simulink model "s_c856m4k"  (R2016b)
settings: Solver=VariableStepAuto  StartTime=0.0  StopTime=10  RelTol=1e-3  EnableMultiTasking=on
undefined symbols (not defined in the file): fft_stages
libraries: xbsIndex_r4 x11811, casper_library_misc x54, casper_library_scopes x5, xps_library x2
(part 10 of 92)

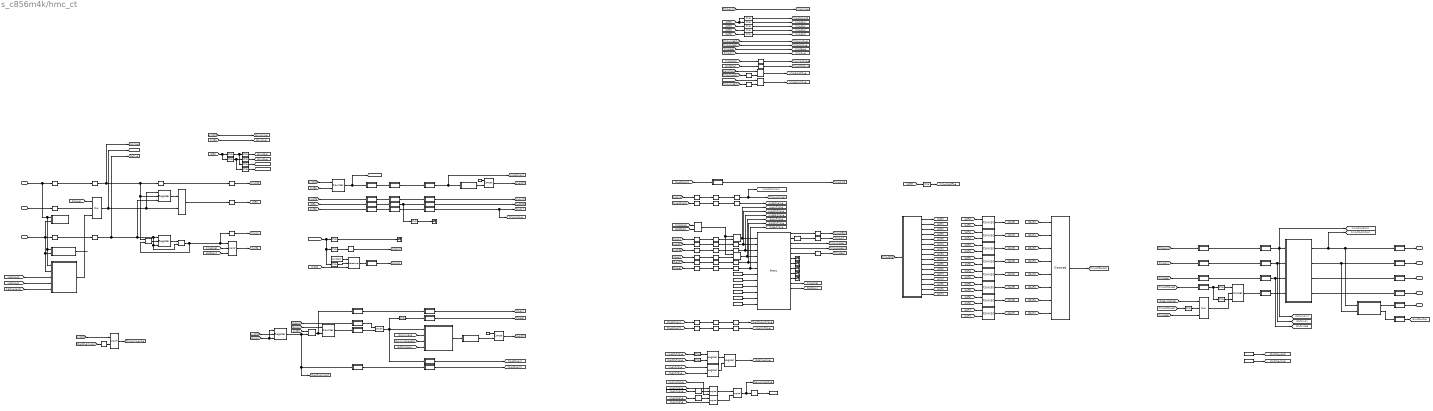
== system s_c856m4k/hmc_ct ==
  note: Sync debugging
  note: Map writes across HMC
      | for performance.
  note: Write two successive words together.
  note: Write is linear.
  note: Read when write switches banks.
  note: Map the output read to collect like channels.
  note: Map writes across HMC
      | for performance.
  note: TVG
  note: Eight parallel channels.
  note: Double buffer the data to form output packets
  note: HMC
  note: Check for _en sync and bank errors
  in_sync : Inport
  in_dv : Inport  Port=2
  in_d128 : Inport  Port=3
  Assertion : Assertion
  Concat{,1..10,12} (12 alike) : xbsIndex_r4/Concat  num_inputs=2  dbl_ovrd=off  block_type=concat
  Concat11 : xbsIndex_r4/Concat  num_inputs=8  dbl_ovrd=off  block_type=concat
  Concat13 : xbsIndex_r4/Concat  num_inputs=3  dbl_ovrd=off  block_type=concat
  Constant : xbsIndex_r4/Constant  const=2^((input_len_bits - 1) + output_len_bits + 1) - 1  gui_display_data_type=Fixed-point  arith_type=Unsigned  n_bits=(input_len_bits - 1) + output_len_bits  bin_pt=0  preci_type=Single  exp_width=8  frac_width=24  explicit_period=on  period=1  equ=P=C  opselect=C  inp2=PCIN>>17  opr=+  inp1=P  carry=CIN  dbl_ovrd=off  block_type=constant
  Constant1 : xbsIndex_r4/Constant  const=0  gui_display_data_type=Boolean  arith_type=Boolean  n_bits=1  bin_pt=0  preci_type=Single  exp_width=8  frac_width=24  explicit_period=on  period=1  equ=P=C  opselect=C  inp2=PCIN>>17  opr=+  inp1=P  carry=CIN  dbl_ovrd=off  block_type=constant
  Constant16 : xbsIndex_r4/Constant  const=384  gui_display_data_type=Fixed-point  arith_type=Unsigned  n_bits=9  bin_pt=0  preci_type=Single  exp_width=8  frac_width=24  explicit_period=on  period=1  equ=P=C  opselect=C  inp2=PCIN>>17  opr=+  inp1=P  carry=CIN  dbl_ovrd=off  block_type=constant
  Constant17 : xbsIndex_r4/Constant  const=128  gui_display_data_type=Fixed-point  arith_type=Unsigned  n_bits=9  bin_pt=0  preci_type=Single  exp_width=8  frac_width=24  explicit_period=on  period=1  equ=P=C  opselect=C  inp2=PCIN>>17  opr=+  inp1=P  carry=CIN  dbl_ovrd=off  block_type=constant
  Constant2 : xbsIndex_r4/Constant  const=0  gui_display_data_type=Fixed-point  arith_type=Unsigned  n_bits=27  bin_pt=0  preci_type=Single  exp_width=8  frac_width=24  explicit_period=on  period=1  equ=P=C  opselect=C  inp2=PCIN>>17  opr=+  inp1=P  carry=CIN  dbl_ovrd=off  block_type=constant
  Constant3 : xbsIndex_r4/Constant  const=0  gui_display_data_type=Fixed-point  arith_type=Unsigned  n_bits=256  bin_pt=0  preci_type=Single  exp_width=8  frac_width=24  explicit_period=on  period=1  equ=P=C  opselect=C  inp2=PCIN>>17  opr=+  inp1=P  carry=CIN  dbl_ovrd=off  block_type=constant
  Constant4 : xbsIndex_r4/Constant  const=0  gui_display_data_type=Fixed-point  arith_type=Unsigned  n_bits=9  bin_pt=0  preci_type=Single  exp_width=8  frac_width=24  explicit_period=on  period=1  equ=P=C  opselect=C  inp2=PCIN>>17  opr=+  inp1=P  carry=CIN  dbl_ovrd=off  block_type=constant
  Constant5 : xbsIndex_r4/Constant  const=0  gui_display_data_type=Boolean  arith_type=Boolean  n_bits=1  bin_pt=0  preci_type=Single  exp_width=8  frac_width=24  explicit_period=on  period=1  equ=P=C  opselect=C  inp2=PCIN>>17  opr=+  inp1=P  carry=CIN  dbl_ovrd=off  block_type=constant
  Constant6 : xbsIndex_r4/Constant  const=0  gui_display_data_type=Fixed-point  arith_type=Unsigned  n_bits=27 - (input_len_bits + output_len_bits)  bin_pt=0  preci_type=Single  exp_width=8  frac_width=24  explicit_period=on  period=1  equ=P=C  opselect=C  inp2=PCIN>>17  opr=+  inp1=P  carry=CIN  dbl_ovrd=off  block_type=constant
  Constant7 : xbsIndex_r4/Constant  const=0  gui_display_data_type=Fixed-point  arith_type=Unsigned  n_bits=27  bin_pt=0  preci_type=Single  exp_width=8  frac_width=24  explicit_period=on  period=1  equ=P=C  opselect=C  inp2=PCIN>>17  opr=+  inp1=P  carry=CIN  dbl_ovrd=off  block_type=constant
  Constant8 : xbsIndex_r4/Constant  const=0  gui_display_data_type=Fixed-point  arith_type=Unsigned  n_bits=27 - (input_len_bits + output_len_bits)  bin_pt=0  preci_type=Single  exp_width=8  frac_width=24  explicit_period=on  period=1  equ=P=C  opselect=C  inp2=PCIN>>17  opr=+  inp1=P  carry=CIN  dbl_ovrd=off  block_type=constant
  Delay{1..2,4..13,16..19,21..23,25..27,30..32,41} (26 alike) : xbsIndex_r4/Delay  rst=off  infoeditControl=Selection of Reset will increase slice count due to use of real FFs and instead of SRLs  en=off  latency=1  reg_retiming=off  dbl_ovrd=off  block_type=delay
      settings: infoedit=Hardware notes: A delay line is a chain, each link of which is an SRL16 or SRL32 followed by a flip-flop.
  Delay{14..15,35,39,42} (5 alike) : xbsIndex_r4/Delay  rst=off  infoeditControl=Selection of Reset will increase slice count due to use of real FFs and instead of SRLs  en=off  latency=2  reg_retiming=off  dbl_ovrd=off  block_type=delay
      settings: infoedit=Hardware notes: A delay line is a chain, each link of which is an SRL16 or SRL32 followed by a flip-flop.
  Delay{3,20,24,28..29,37..38,40} (8 alike) : xbsIndex_r4/Delay  rst=off  infoeditControl=Selection of Reset will increase slice count due to use of real FFs and instead of SRLs  en=off  latency=5  reg_retiming=off  dbl_ovrd=off  block_type=delay
      settings: infoedit=Hardware notes: A delay line is a chain, each link of which is an SRL16 or SRL32 followed by a flip-flop.
  Delay33 : xbsIndex_r4/Delay  rst=off  infoeditControl=Selection of Reset will increase slice count due to use of real FFs and instead of SRLs  en=off  latency=4  reg_retiming=off  dbl_ovrd=off  block_type=delay
      settings: infoedit=Hardware notes: A delay line is a chain, each link of which is an SRL16 or SRL32 followed by a flip-flop.
  Delay34 : xbsIndex_r4/Delay  rst=off  infoeditControl=Selection of Reset will increase slice count due to use of real FFs and instead of SRLs  en=off  latency=4  reg_retiming=off  dbl_ovrd=off  block_type=delay
      settings: infoedit=Hardware notes: A delay line is a chain, each link of which is an SRL16 or SRL32 followed by a flip-flop.
  Delay36 : xbsIndex_r4/Delay  rst=off  infoeditControl=Selection of Reset will increase slice count due to use of real FFs and instead of SRLs  en=off  latency=4  reg_retiming=off  dbl_ovrd=off  block_type=delay
      settings: infoedit=Hardware notes: A delay line is a chain, each link of which is an SRL16 or SRL32 followed by a flip-flop.
  Inverter{,1..2,4..6} (6 alike) : xbsIndex_r4/Inverter  en=off  latency=0  dbl_ovrd=off  block_type=inv
  Inverter3 : xbsIndex_r4/Inverter  en=off  latency=1  dbl_ovrd=off  block_type=inv
  Logical : xbsIndex_r4/Logical  logical_function=AND  inputs=2  en=off  latency=0  precision=Full  arith_type=Unsigned  n_bits=16  bin_pt=0  align_bp=on  dbl_ovrd=off  block_type=logical
  Logical1 : xbsIndex_r4/Logical  logical_function=AND  inputs=2  en=off  latency=1  precision=User Defined  arith_type=Boolean  n_bits=1  bin_pt=0  align_bp=on  dbl_ovrd=off  block_type=logical
  Logical10 : xbsIndex_r4/Logical  logical_function=OR  inputs=2  en=off  latency=0  precision=Full  arith_type=Unsigned  n_bits=16  bin_pt=0  align_bp=on  dbl_ovrd=off  block_type=logical
  Logical{5,7,11,13} (4 alike) : xbsIndex_r4/Logical  logical_function=AND  inputs=2  en=off  latency=5  precision=Full  arith_type=Unsigned  n_bits=16  bin_pt=0  align_bp=on  dbl_ovrd=off  block_type=logical
  Logical12 : xbsIndex_r4/Logical  logical_function=AND  inputs=2  en=off  latency=1  precision=User Defined  arith_type=Boolean  n_bits=1  bin_pt=0  align_bp=on  dbl_ovrd=off  block_type=logical
  Logical14 : xbsIndex_r4/Logical  logical_function=OR  inputs=2  en=off  latency=5  precision=Full  arith_type=Unsigned  n_bits=16  bin_pt=0  align_bp=on  dbl_ovrd=off  block_type=logical
  Logical15 : xbsIndex_r4/Logical  logical_function=AND  inputs=2  en=off  latency=2  precision=Full  arith_type=Unsigned  n_bits=16  bin_pt=0  align_bp=on  dbl_ovrd=off  block_type=logical
  Logical2 : xbsIndex_r4/Logical  logical_function=OR  inputs=2  en=off  latency=0  precision=Full  arith_type=Unsigned  n_bits=16  bin_pt=0  align_bp=on  dbl_ovrd=off  block_type=logical
  Logical3 : xbsIndex_r4/Logical  logical_function=AND  inputs=2  en=off  latency=0  precision=Full  arith_type=Unsigned  n_bits=16  bin_pt=0  align_bp=on  dbl_ovrd=off  block_type=logical
  Logical4 : xbsIndex_r4/Logical  logical_function=AND  inputs=2  en=off  latency=1  precision=Full  arith_type=Unsigned  n_bits=16  bin_pt=0  align_bp=on  dbl_ovrd=off  block_type=logical
  Logical6 : xbsIndex_r4/Logical  logical_function=AND  inputs=2  en=on  latency=5  precision=Full  arith_type=Unsigned  n_bits=16  bin_pt=0  align_bp=on  dbl_ovrd=off  block_type=logical
  Logical8 : xbsIndex_r4/Logical  logical_function=AND  inputs=2  en=off  latency=0  precision=Full  arith_type=Unsigned  n_bits=16  bin_pt=0  align_bp=on  dbl_ovrd=off  block_type=logical
  Logical9 : xbsIndex_r4/Logical  logical_function=AND  inputs=3  en=off  latency=2  precision=Full  arith_type=Unsigned  n_bits=16  bin_pt=0  align_bp=on  dbl_ovrd=off  block_type=logical
  Mux : xbsIndex_r4/Mux  inputs=2  en=off  latency=2  precision=Full  arith_type=Unsigned  n_bits=16  bin_pt=14  quantization=Truncate  overflow=Wrap  dbl_ovrd=off  block_type=mux
  Mux3 : xbsIndex_r4/Mux  inputs=2  en=off  latency=2  precision=Full  arith_type=Unsigned  n_bits=16  bin_pt=14  quantization=Truncate  overflow=Wrap  dbl_ovrd=off  block_type=mux
  Register : xbsIndex_r4/Register  init=0  rst=on  en=on  dbl_ovrd=off  block_type=register
  Relational1 : xbsIndex_r4/Relational  mode=a=b  op_type=Bool  en=on  latency=1  dbl_ovrd=off  block_type=relational
  Slice : xbsIndex_r4/Slice  nbits=12  boolean_output=off  mode=Lower Bit Location + Width  bit1=0  base1=MSB of Input  bit0=0  base0=LSB of Input  dbl_ovrd=off  block_type=slice
  Slice1 : xbsIndex_r4/Slice  nbits=9  boolean_output=off  mode=Lower Bit Location + Width  bit1=0  base1=MSB of Input  bit0=0  base0=LSB of Input  dbl_ovrd=off  block_type=slice
  Slice12 : xbsIndex_r4/Slice  nbits=1  boolean_output=on  mode=Lower Bit Location + Width  bit1=0  base1=MSB of Input  bit0=input_len_bits - 1 + output_len_bits  base0=LSB of Input  dbl_ovrd=off  block_type=slice
  Slice13 : xbsIndex_r4/Slice  nbits=1  boolean_output=on  mode=Lower Bit Location + Width  bit1=0  base1=MSB of Input  bit0=input_len_bits - 1 + output_len_bits  base0=LSB of Input  dbl_ovrd=off  block_type=slice
  Slice{2..5} (4 alike) : xbsIndex_r4/Slice  nbits=input_len_bits + 2  boolean_output=off  mode=Lower Bit Location + Width  bit1=0  base1=MSB of Input  bit0=0  base0=LSB of Input  dbl_ovrd=off  block_type=slice
  Slice6 : xbsIndex_r4/Slice  nbits=input_len_bits + 2  boolean_output=on  mode=Upper Bit Location + Width  bit1=0  base1=MSB of Input  bit0=0  base0=LSB of Input  dbl_ovrd=off  block_type=slice
  Terminator{1,16,20..24} (7 alike) : Terminator
  bank : xbsIndex_r4/Slice  nbits=1  boolean_output=on  mode=Upper Bit Location + Width  bit1=0  base1=MSB of Input  bit0=0  base0=LSB of Input  dbl_ovrd=off  block_type=slice
  bank1 : xbsIndex_r4/Slice  nbits=12  boolean_output=off  mode=Upper Bit Location + Width  bit1=-4  base1=MSB of Input  bit0=0  base0=LSB of Input  dbl_ovrd=off  block_type=slice
  bank2 : xbsIndex_r4/Slice  nbits=12  boolean_output=off  mode=Upper Bit Location + Width  bit1=-4  base1=MSB of Input  bit0=128  base0=LSB of Input  dbl_ovrd=off  block_type=slice
  bank3 : xbsIndex_r4/Slice  nbits=12  boolean_output=off  mode=Upper Bit Location + Width  bit1=-4  base1=MSB of Input  bit0=128  base0=LSB of Input  dbl_ovrd=off  block_type=slice
  bank4 : xbsIndex_r4/Slice  nbits=128  boolean_output=off  mode=Lower Bit Location + Width  bit1=0  base1=MSB of Input  bit0=128  base0=LSB of Input  dbl_ovrd=off  block_type=slice
  bank5 : xbsIndex_r4/Slice  nbits=128  boolean_output=off  mode=Lower Bit Location + Width  bit1=0  base1=MSB of Input  bit0=0  base0=LSB of Input  dbl_ovrd=off  block_type=slice
  bank6 : xbsIndex_r4/Slice  nbits=12  boolean_output=on  mode=Upper Bit Location + Width  bit1=0  base1=MSB of Input  bit0=128  base0=LSB of Input  dbl_ovrd=off  block_type=slice
  bank7 : xbsIndex_r4/Slice  nbits=12  boolean_output=on  mode=Upper Bit Location + Width  bit1=0  base1=MSB of Input  bit0=128  base0=LSB of Input  dbl_ovrd=off  block_type=slice
  bus_expand1 : Subsystem  AncestorBlock=casper_library_flow_control/bus_expand  mask(bus_expand){mode=divisions of equal size, outputNum=16, outputWidth=16, outputBinaryPt=0, outputArithmeticType=0, show_format=off, outputToWorkspace=off, variablePrefix=out, outputToModelAsWell=on}
      mask prompts: outputNum "Number of outputs:"; outputWidth "Output width:"; outputBinaryPt "Output binary point position:"; outputArithmeticType "Output arithmetic type (ufix=0, fix=1, bool=2):"; show_format "Print format string?"; outputToWorkspace "Output to workspace?"; variablePrefix "Variable name prefix:"; outputToModelAsWell "Output to model as well?"
      mask help:
      | Expands a 'bus' made using a bus_create or Xilinx
      | concat block.
      | The input will be divided into the specified number
      | of outputs with the specified arithmetic types.
      | Divisions are made from most significant bit.
      mask init: same as s_c856m4k/bus_expand
      settings: AttributesFormatString=16 outputs
      mask TypeOptions mode: divisions of equal size | divisions of arbitrary size
      mask Callback mode: bus_expand_callback();
      mask Callback outputWidth: bus_expand_callback();
      mask Callback outputToWorkspace: bus_expand_callback();
  convert_rd_en4 : xbsIndex_r4/Convert  gui_display_data_type=Boolean  arith_type=Boolean  n_bits=128  bin_pt=0  float_type=Single  exp_bits=8  fraction_bits=24  quantization=Truncate  overflow=Wrap  en=off  latency=0  pipeline=off  dbl_ovrd=off  block_type=convert
      settings: xl_area=[0, 0, 0, 0, 0, 0, 0]
  edge_detect1 : Subsystem  AncestorBlock=casper_library_misc/edge_detect  mask(edge_detect){edge=Rising, polarity=Active High, x_in=[0 0.08 0.08 0.16 0.16 0.24 0.24 0.32 0.32 0.4], y_in=[-1 -1  1  1  1  1  1  1  1  1], x_out=[0.6 0.68 0.68 0.76 0.76 0.84 0.84 0.92 0.92 1], y_out=[-1 -1  1  1 -1 -1 -1 -1 -1 -1]}
      mask prompts: edge "Edge Type"; polarity "Output Polarity"; x_in "Input X Positions"; y_in "Input Y Positions"; x_out "Output X Positions"; y_out "Output Y Positions"
      mask help: Output is active for one-cycle after each edge of the specified type (i.e. rising, falling or both).
      mask init: same as s_c856m4k/edge_detect1
      settings: AttributesFormatString=|
      | rising edges
      | active high
      mask Help: Output is active for one-cycle after each edge of the specified type (i.e. rising, falling, or both).  Latency is zero.
      mask TypeOptions edge: Rising | Falling | Both
      mask TypeOptions polarity: Active High | Active Low
      mask Display:
      | plot(x_in_num,0.5+y_in_num*0.2);
      | plot(x_out_num,0.5+y_out_num*0.2);
  edge_detect2 : Subsystem  AncestorBlock=casper_library_misc/edge_detect  mask(edge_detect){edge=Rising, polarity=Active High, x_in=[0 0.08 0.08 0.16 0.16 0.24 0.24 0.32 0.32 0.4], y_in=[-1 -1  1  1  1  1  1  1  1  1], x_out=[0.6 0.68 0.68 0.76 0.76 0.84 0.84 0.92 0.92 1], y_out=[-1 -1  1  1 -1 -1 -1 -1 -1 -1]}
      mask prompts: edge "Edge Type"; polarity "Output Polarity"; x_in "Input X Positions"; y_in "Input Y Positions"; x_out "Output X Positions"; y_out "Output Y Positions"
      mask help: Output is active for one-cycle after each edge of the specified type (i.e. rising, falling or both).
      mask init: same as s_c856m4k/edge_detect1
      settings: AttributesFormatString=|
      | rising edges
      | active high
      mask Help: Output is active for one-cycle after each edge of the specified type (i.e. rising, falling, or both).  Latency is zero.
      mask TypeOptions edge: Rising | Falling | Both
      mask TypeOptions polarity: Active High | Active Low
      mask Display:
      | plot(x_in_num,0.5+y_in_num*0.2);
      | plot(x_out_num,0.5+y_out_num*0.2);
  hmc : xps_library/hmc  Tag=xps:hmc  mez=0  sim_depth=(input_len_bits-1) + output_len_bits + 1  sim_latency=5  sim_rand=on
  hmc_addr_opt : Subsystem
  hmc_addr_opt1 : Subsystem
  last_tag2 : xbsIndex_r4/Register  init=0  rst=on  en=on  dbl_ovrd=off  block_type=register
  make_interleaved_freqs : Subsystem  mask{chan_bits=12, xeng_bits=4}
      mask prompts: chan_bits "Number of channels (2^?)"; xeng_bits "Number of x-engines (2^?)"
  obuf : Subsystem  mask{output_vec_bits=output_len_bits, pkt_buffer_latency=10, omux_latency=15}
      mask prompts: output_vec_bits "CT output vector bits"; pkt_buffer_latency "Output buffer latency"; omux_latency "Output mux latency"
  prev_word : xbsIndex_r4/Register  init=0  rst=on  en=on  dbl_ovrd=off  block_type=register
  rd_addr_ctr : xbsIndex_r4/Counter  cnt_type=Free Running  cnt_to=Inf  operation=Up  start_count=0  cnt_by_val=1  arith_type=Unsigned  n_bits=input_len_bits - 1 + output_len_bits  bin_pt=0  load_pin=off  rst=on  en=on  explicit_period=on  period=1  use_behavioral_HDL=off  implementation=Fabric  dbl_ovrd=off  block_type=counter
  read_map_gen_interleave : Subsystem  mask{in_vec_bits=input_len_bits - 1, out_vec_bits=output_len_bits}
      mask prompts: in_vec_bits "Input vector bits"; out_vec_bits "Output vector bits"
      mask init:
      | vec_len = 2^in_vec_bits * 2^out_vec_bits;
      | mystr = sprintf('2^%i x 2^%i = %i', in_vec_bits, out_vec_bits, vec_len);
      | set_param(gcb, 'AttributesFormatString', mystr);
      settings: AttributesFormatString=2^9 x 2^8 = 131072
  spectrum_ctr : xbsIndex_r4/Slice  nbits=1  boolean_output=off  mode=Two Bit Locations  bit1=-1  base1=MSB of Input  bit0=input_len_bits - 1  base0=LSB of Input  dbl_ovrd=off  block_type=slice
  spectrum_ctr1 : xbsIndex_r4/Slice  nbits=1  boolean_output=off  mode=Two Bit Locations  bit1=-1  base1=MSB of Input  bit0=0  base0=LSB of Input  dbl_ovrd=off  block_type=slice
  spectrum_ctr2 : xbsIndex_r4/Slice  nbits=256 - (32 + 9)  boolean_output=off  mode=Lower Bit Location + Width  bit1=-1  base1=MSB of Input  bit0=32 + 9  base0=LSB of Input  dbl_ovrd=off  block_type=slice
  spectrum_ctr3 : xbsIndex_r4/Slice  nbits=32  boolean_output=off  mode=Lower Bit Location + Width  bit1=-1  base1=MSB of Input  bit0=0  base0=LSB of Input  dbl_ovrd=off  block_type=slice
  spectrum_ctr4 : xbsIndex_r4/Slice  nbits=9  boolean_output=off  mode=Lower Bit Location + Width  bit1=-1  base1=MSB of Input  bit0=32  base0=LSB of Input  dbl_ovrd=off  block_type=slice
  tvg_data_gen : Subsystem
  tvg_data_gen_oneshot : Subsystem
      mask Display:
      | color('red');
      | disp('ONE SHOT!!');
      | % color('green');
      | % port_label('input', 1, 'dv')
      | % color('red');
      | % port_label('output', 1, 'err')
  tvg_data_tone_gen : Subsystem
  waddr : xbsIndex_r4/Counter  cnt_type=Free Running  cnt_to=Inf  operation=Up  start_count=0  cnt_by_val=1  arith_type=Unsigned  n_bits=input_len_bits + output_len_bits  bin_pt=0  load_pin=off  rst=on  en=on  explicit_period=on  period=1  use_behavioral_HDL=off  implementation=Fabric  dbl_ovrd=off  block_type=counter
  we_delay1 : Subsystem  AncestorBlock=casper_library_delays/pipeline  mask(pipeline){latency=2}
      mask help:
      | An explicitly laid-out delay line to avoid mapping to SRL16s
      | for use in pipelining to help achieve timing closure.
      mask init:
      | pipeline_init(gcb,'latency',latency);
      settings: AttributesFormatString=Latency = %<latency>
      mask Display:
      | port_label('input', 1, 'd');
      | port_label('output', 1, 'q');
      | disp(['Z^-', num2str(latency)]);
  we_delay10 : Subsystem  AncestorBlock=casper_library_delays/pipeline  mask(pipeline){latency=2}
      mask help:
      | An explicitly laid-out delay line to avoid mapping to SRL16s
      | for use in pipelining to help achieve timing closure.
      mask init:
      | pipeline_init(gcb,'latency',latency);
      settings: AttributesFormatString=Latency = %<latency>
      mask Display:
      | port_label('input', 1, 'd');
      | port_label('output', 1, 'q');
      | disp(['Z^-', num2str(latency)]);
  we_delay11 : Subsystem  AncestorBlock=casper_library_delays/pipeline  mask(pipeline){latency=2}
      mask help:
      | An explicitly laid-out delay line to avoid mapping to SRL16s
      | for use in pipelining to help achieve timing closure.
      mask init:
      | pipeline_init(gcb,'latency',latency);
      settings: AttributesFormatString=Latency = %<latency>
      mask Display:
      | port_label('input', 1, 'd');
      | port_label('output', 1, 'q');
      | disp(['Z^-', num2str(latency)]);
  we_delay12 : Subsystem  AncestorBlock=casper_library_delays/pipeline  mask(pipeline){latency=2}
      mask help:
      | An explicitly laid-out delay line to avoid mapping to SRL16s
      | for use in pipelining to help achieve timing closure.
      mask init:
      | pipeline_init(gcb,'latency',latency);
      settings: AttributesFormatString=Latency = %<latency>
      mask Display:
      | port_label('input', 1, 'd');
      | port_label('output', 1, 'q');
      | disp(['Z^-', num2str(latency)]);
  we_delay13 : Subsystem  AncestorBlock=casper_library_delays/pipeline  mask(pipeline){latency=1}
      mask help:
      | An explicitly laid-out delay line to avoid mapping to SRL16s
      | for use in pipelining to help achieve timing closure.
      mask init:
      | pipeline_init(gcb,'latency',latency);
      settings: AttributesFormatString=Latency = %<latency>
      mask Display:
      | port_label('input', 1, 'd');
      | port_label('output', 1, 'q');
      | disp(['Z^-', num2str(latency)]);
  we_delay14 : Subsystem  AncestorBlock=casper_library_delays/pipeline  mask(pipeline){latency=3}
      mask help:
      | An explicitly laid-out delay line to avoid mapping to SRL16s
      | for use in pipelining to help achieve timing closure.
      mask init:
      | pipeline_init(gcb,'latency',latency);
      settings: AttributesFormatString=Latency = %<latency>
      mask Display:
      | port_label('input', 1, 'd');
      | port_label('output', 1, 'q');
      | disp(['Z^-', num2str(latency)]);
  we_delay15 : Subsystem  AncestorBlock=casper_library_delays/pipeline  mask(pipeline){latency=3}
      mask help:
      | An explicitly laid-out delay line to avoid mapping to SRL16s
      | for use in pipelining to help achieve timing closure.
      mask init:
      | pipeline_init(gcb,'latency',latency);
      settings: AttributesFormatString=Latency = %<latency>
      mask Display:
      | port_label('input', 1, 'd');
      | port_label('output', 1, 'q');
      | disp(['Z^-', num2str(latency)]);
  we_delay16 : Subsystem  AncestorBlock=casper_library_delays/pipeline  mask(pipeline){latency=3}
      mask help:
      | An explicitly laid-out delay line to avoid mapping to SRL16s
      | for use in pipelining to help achieve timing closure.
      mask init:
      | pipeline_init(gcb,'latency',latency);
      settings: AttributesFormatString=Latency = %<latency>
      mask Display:
      | port_label('input', 1, 'd');
      | port_label('output', 1, 'q');
      | disp(['Z^-', num2str(latency)]);
  we_delay17 : Subsystem  AncestorBlock=casper_library_delays/pipeline  mask(pipeline){latency=3}
      mask help:
      | An explicitly laid-out delay line to avoid mapping to SRL16s
      | for use in pipelining to help achieve timing closure.
      mask init:
      | pipeline_init(gcb,'latency',latency);
      settings: AttributesFormatString=Latency = %<latency>
      mask Display:
      | port_label('input', 1, 'd');
      | port_label('output', 1, 'q');
      | disp(['Z^-', num2str(latency)]);
  we_delay18 : Subsystem  AncestorBlock=casper_library_delays/pipeline  mask(pipeline){latency=3}
      mask help:
      | An explicitly laid-out delay line to avoid mapping to SRL16s
      | for use in pipelining to help achieve timing closure.
      mask init:
      | pipeline_init(gcb,'latency',latency);
      settings: AttributesFormatString=Latency = %<latency>
      mask Display:
      | port_label('input', 1, 'd');
      | port_label('output', 1, 'q');
      | disp(['Z^-', num2str(latency)]);
  we_delay19 : Subsystem  AncestorBlock=casper_library_delays/pipeline  mask(pipeline){latency=3}
      mask help:
      | An explicitly laid-out delay line to avoid mapping to SRL16s
      | for use in pipelining to help achieve timing closure.
      mask init:
      | pipeline_init(gcb,'latency',latency);
      settings: AttributesFormatString=Latency = %<latency>
      mask Display:
      | port_label('input', 1, 'd');
      | port_label('output', 1, 'q');
      | disp(['Z^-', num2str(latency)]);
  we_delay2 : Subsystem  AncestorBlock=casper_library_delays/pipeline  mask(pipeline){latency=2}
      mask help:
      | An explicitly laid-out delay line to avoid mapping to SRL16s
      | for use in pipelining to help achieve timing closure.
      mask init:
      | pipeline_init(gcb,'latency',latency);
      settings: AttributesFormatString=Latency = %<latency>
      mask Display:
      | port_label('input', 1, 'd');
      | port_label('output', 1, 'q');
      | disp(['Z^-', num2str(latency)]);
  we_delay20 : Subsystem  AncestorBlock=casper_library_delays/pipeline  mask(pipeline){latency=3}
      mask help:
      | An explicitly laid-out delay line to avoid mapping to SRL16s
      | for use in pipelining to help achieve timing closure.
      mask init:
      | pipeline_init(gcb,'latency',latency);
      settings: AttributesFormatString=Latency = %<latency>
      mask Display:
      | port_label('input', 1, 'd');
      | port_label('output', 1, 'q');
      | disp(['Z^-', num2str(latency)]);
  we_delay21 : Subsystem  AncestorBlock=casper_library_delays/pipeline  mask(pipeline){latency=1}
      mask help:
      | An explicitly laid-out delay line to avoid mapping to SRL16s
      | for use in pipelining to help achieve timing closure.
      mask init:
      | pipeline_init(gcb,'latency',latency);
      settings: AttributesFormatString=Latency = %<latency>
      mask Display:
      | port_label('input', 1, 'd');
      | port_label('output', 1, 'q');
      | disp(['Z^-', num2str(latency)]);
  we_delay22 : Subsystem  AncestorBlock=casper_library_delays/pipeline  mask(pipeline){latency=15}
      mask help:
      | An explicitly laid-out delay line to avoid mapping to SRL16s
      | for use in pipelining to help achieve timing closure.
      mask init:
      | pipeline_init(gcb,'latency',latency);
      settings: AttributesFormatString=Latency = %<latency>
      mask Display:
      | port_label('input', 1, 'd');
      | port_label('output', 1, 'q');
      | disp(['Z^-', num2str(latency)]);
  we_delay23 : Subsystem  AncestorBlock=casper_library_delays/pipeline  mask(pipeline){latency=15}
      mask help:
      | An explicitly laid-out delay line to avoid mapping to SRL16s
      | for use in pipelining to help achieve timing closure.
      mask init:
      | pipeline_init(gcb,'latency',latency);
      settings: AttributesFormatString=Latency = %<latency>
      mask Display:
      | port_label('input', 1, 'd');
      | port_label('output', 1, 'q');
      | disp(['Z^-', num2str(latency)]);
  we_delay24 : Subsystem  AncestorBlock=casper_library_delays/pipeline  mask(pipeline){latency=15}
      mask help:
      | An explicitly laid-out delay line to avoid mapping to SRL16s
      | for use in pipelining to help achieve timing closure.
      mask init:
      | pipeline_init(gcb,'latency',latency);
      settings: AttributesFormatString=Latency = %<latency>
      mask Display:
      | port_label('input', 1, 'd');
      | port_label('output', 1, 'q');
      | disp(['Z^-', num2str(latency)]);
  we_delay25 : Subsystem  AncestorBlock=casper_library_delays/pipeline  mask(pipeline){latency=15}
      mask help:
      | An explicitly laid-out delay line to avoid mapping to SRL16s
      | for use in pipelining to help achieve timing closure.
      mask init:
      | pipeline_init(gcb,'latency',latency);
      settings: AttributesFormatString=Latency = %<latency>
      mask Display:
      | port_label('input', 1, 'd');
      | port_label('output', 1, 'q');
      | disp(['Z^-', num2str(latency)]);
  we_delay26 : Subsystem  AncestorBlock=casper_library_delays/pipeline  mask(pipeline){latency=15}
      mask help:
      | An explicitly laid-out delay line to avoid mapping to SRL16s
      | for use in pipelining to help achieve timing closure.
      mask init:
      | pipeline_init(gcb,'latency',latency);
      settings: AttributesFormatString=Latency = %<latency>
      mask Display:
      | port_label('input', 1, 'd');
      | port_label('output', 1, 'q');
      | disp(['Z^-', num2str(latency)]);
  we_delay27 : Subsystem  AncestorBlock=casper_library_delays/pipeline  mask(pipeline){latency=15}
      mask help:
      | An explicitly laid-out delay line to avoid mapping to SRL16s
      | for use in pipelining to help achieve timing closure.
      mask init:
      | pipeline_init(gcb,'latency',latency);
      settings: AttributesFormatString=Latency = %<latency>
      mask Display:
      | port_label('input', 1, 'd');
      | port_label('output', 1, 'q');
      | disp(['Z^-', num2str(latency)]);
  we_delay28 : Subsystem  AncestorBlock=casper_library_delays/pipeline  mask(pipeline){latency=15}
      mask help:
      | An explicitly laid-out delay line to avoid mapping to SRL16s
      | for use in pipelining to help achieve timing closure.
      mask init:
      | pipeline_init(gcb,'latency',latency);
      settings: AttributesFormatString=Latency = %<latency>
      mask Display:
      | port_label('input', 1, 'd');
      | port_label('output', 1, 'q');
      | disp(['Z^-', num2str(latency)]);
  we_delay29 : Subsystem  AncestorBlock=casper_library_delays/pipeline  mask(pipeline){latency=15}
      mask help:
      | An explicitly laid-out delay line to avoid mapping to SRL16s
      | for use in pipelining to help achieve timing closure.
      mask init:
      | pipeline_init(gcb,'latency',latency);
      settings: AttributesFormatString=Latency = %<latency>
      mask Display:
      | port_label('input', 1, 'd');
      | port_label('output', 1, 'q');
      | disp(['Z^-', num2str(latency)]);
  we_delay3 : Subsystem  AncestorBlock=casper_library_delays/pipeline  mask(pipeline){latency=2}
      mask help:
      | An explicitly laid-out delay line to avoid mapping to SRL16s
      | for use in pipelining to help achieve timing closure.
      mask init:
      | pipeline_init(gcb,'latency',latency);
      settings: AttributesFormatString=Latency = %<latency>
      mask Display:
      | port_label('input', 1, 'd');
      | port_label('output', 1, 'q');
      | disp(['Z^-', num2str(latency)]);
  we_delay30 : Subsystem  AncestorBlock=casper_library_delays/pipeline  mask(pipeline){latency=3}
      mask help:
      | An explicitly laid-out delay line to avoid mapping to SRL16s
      | for use in pipelining to help achieve timing closure.
      mask init:
      | pipeline_init(gcb,'latency',latency);
      settings: AttributesFormatString=Latency = %<latency>
      mask Display:
      | port_label('input', 1, 'd');
      | port_label('output', 1, 'q');
      | disp(['Z^-', num2str(latency)]);
  we_delay31 : Subsystem  AncestorBlock=casper_library_delays/pipeline  mask(pipeline){latency=1}
      mask help:
      | An explicitly laid-out delay line to avoid mapping to SRL16s
      | for use in pipelining to help achieve timing closure.
      mask init:
      | pipeline_init(gcb,'latency',latency);
      settings: AttributesFormatString=Latency = %<latency>
      mask Display:
      | port_label('input', 1, 'd');
      | port_label('output', 1, 'q');
      | disp(['Z^-', num2str(latency)]);
  we_delay32 : Subsystem  AncestorBlock=casper_library_delays/pipeline  mask(pipeline){latency=1}
      mask help:
      | An explicitly laid-out delay line to avoid mapping to SRL16s
      | for use in pipelining to help achieve timing closure.
      mask init:
      | pipeline_init(gcb,'latency',latency);
      settings: AttributesFormatString=Latency = %<latency>
      mask Display:
      | port_label('input', 1, 'd');
      | port_label('output', 1, 'q');
      | disp(['Z^-', num2str(latency)]);
  we_delay33 : Subsystem  AncestorBlock=casper_library_delays/pipeline  mask(pipeline){latency=2}
      mask help:
      | An explicitly laid-out delay line to avoid mapping to SRL16s
      | for use in pipelining to help achieve timing closure.
      mask init:
      | pipeline_init(gcb,'latency',latency);
      settings: AttributesFormatString=Latency = %<latency>
      mask Display:
      | port_label('input', 1, 'd');
      | port_label('output', 1, 'q');
      | disp(['Z^-', num2str(latency)]);
  we_delay34 : Subsystem  AncestorBlock=casper_library_delays/pipeline  mask(pipeline){latency=2}
      mask help:
      | An explicitly laid-out delay line to avoid mapping to SRL16s
      | for use in pipelining to help achieve timing closure.
      mask init:
      | pipeline_init(gcb,'latency',latency);
      settings: AttributesFormatString=Latency = %<latency>
      mask Display:
      | port_label('input', 1, 'd');
      | port_label('output', 1, 'q');
      | disp(['Z^-', num2str(latency)]);
  we_delay4 : Subsystem  AncestorBlock=casper_library_delays/pipeline  mask(pipeline){latency=2}
      mask help:
      | An explicitly laid-out delay line to avoid mapping to SRL16s
      | for use in pipelining to help achieve timing closure.
      mask init:
      | pipeline_init(gcb,'latency',latency);
      settings: AttributesFormatString=Latency = %<latency>
      mask Display:
      | port_label('input', 1, 'd');
      | port_label('output', 1, 'q');
      | disp(['Z^-', num2str(latency)]);
  we_delay5 : Subsystem  AncestorBlock=casper_library_delays/pipeline  mask(pipeline){latency=2}
      mask help:
      | An explicitly laid-out delay line to avoid mapping to SRL16s
      | for use in pipelining to help achieve timing closure.
      mask init:
      | pipeline_init(gcb,'latency',latency);
      settings: AttributesFormatString=Latency = %<latency>
      mask Display:
      | port_label('input', 1, 'd');
      | port_label('output', 1, 'q');
      | disp(['Z^-', num2str(latency)]);
  we_delay6 : Subsystem  AncestorBlock=casper_library_delays/pipeline  mask(pipeline){latency=2}
      mask help:
      | An explicitly laid-out delay line to avoid mapping to SRL16s
      | for use in pipelining to help achieve timing closure.
      mask init:
      | pipeline_init(gcb,'latency',latency);
      settings: AttributesFormatString=Latency = %<latency>
      mask Display:
      | port_label('input', 1, 'd');
      | port_label('output', 1, 'q');
      | disp(['Z^-', num2str(latency)]);
  we_delay7 : Subsystem  AncestorBlock=casper_library_delays/pipeline  mask(pipeline){latency=2}
      mask help:
      | An explicitly laid-out delay line to avoid mapping to SRL16s
      | for use in pipelining to help achieve timing closure.
      mask init:
      | pipeline_init(gcb,'latency',latency);
      settings: AttributesFormatString=Latency = %<latency>
      mask Display:
      | port_label('input', 1, 'd');
      | port_label('output', 1, 'q');
      | disp(['Z^-', num2str(latency)]);
  we_delay8 : Subsystem  AncestorBlock=casper_library_delays/pipeline  mask(pipeline){latency=2}
      mask help:
      | An explicitly laid-out delay line to avoid mapping to SRL16s
      | for use in pipelining to help achieve timing closure.
      mask init:
      | pipeline_init(gcb,'latency',latency);
      settings: AttributesFormatString=Latency = %<latency>
      mask Display:
      | port_label('input', 1, 'd');
      | port_label('output', 1, 'q');
      | disp(['Z^-', num2str(latency)]);
  we_delay9 : Subsystem  AncestorBlock=casper_library_delays/pipeline  mask(pipeline){latency=2}
      mask help:
      | An explicitly laid-out delay line to avoid mapping to SRL16s
      | for use in pipelining to help achieve timing closure.
      mask init:
      | pipeline_init(gcb,'latency',latency);
      settings: AttributesFormatString=Latency = %<latency>
      mask Display:
      | port_label('input', 1, 'd');
      | port_label('output', 1, 'q');
      | disp(['Z^-', num2str(latency)]);
  out_sync : Outport
  out_dv : Outport  Port=2
  out_d256 : Outport  Port=3
  pkt_start : Outport  Port=4
  freq_id : Outport  Port=5
  tag scope: ct_bank_error_g=global, ct_en_sync_error_g=global, ct_in_d0_g=global, ct_in_d0_msb_g=global, ct_in_d1_g=global, ct_in_d1_msb_g=global, ct_in_dv_g=global, ct_in_sync_g=global, cthmc_sync_err0_g=global, d256=global, dv256=global, hmc_d0_0=global, hmc_d0_0_msb=global, hmc_d0_1=global, hmc_d0_2=global, hmc_d0_3=global, hmc_dv=global, hmc_dv_g=global, hmc_err_rdrdy_g=global, hmc_err_wrrdy_g=global, hmc_init_done_g=global, hmc_out_p0f0_g=global, hmc_postokay_g=global, hmc_rd_rdy_g=global, hmc_sync_g=global, hmc_tag_g=global, hmc_wr_dv_g=global, hmc_wr_rdy_g=global, hmc_wr_sync_g=global, obuf_in_dv=global, obuf_in_sync=global, obuf_in_tag=global, obuf_trig_lower=global, obuf_trig_upper=global, qt_d128_g=global, qt_dv_g=global, qt_sync_g=global, raw_freq_ctr_g=global, rd_addr_final_g=global, rd_addr_raw_final_g=global, rd_arm_final_g=global, rd_en_final_g=global, rd_tag_final_g=global, sync256=global, sync_ctrs_hmc_in=global, sync_ctrs_obuf_in=global, sync_ctrs_obuf_out=global, wr_addr_final_g=global, wr_addr_raw_g=global, wr_data_final_g=global, wr_en_final_g=global
  wires:
  Logical15/1 -> [cthmc_sync_err0_g]
  Inverter6/1 -> Logical15/2
  [sync256] -> Logical15/1
  [rd_addr_arm_raw] -> Inverter6/1
  edge_detect1/1(out) -> [hmc_sync]
  [rd_addr_arm] -> edge_detect1/1(in)
  we_delay34/1(q) -> [raw_freq_ctr_g]
  make_interleaved_freqs/2(raw_ctr) -> we_delay34/1(d)
  Delay40/1 -> [sync_ctrs_hmc_in], [hmc_wr_sync_g]
  Slice6/1 -> [hmc_d0_0_msb]
  bank7/1 -> [ct_in_d1_msb_g]
  bank6/1 -> [ct_in_d0_msb_g]
  tvg_data_gen/1(d128) -> ?
  Delay36/1 -> Delay35/1
  Delay33/1 -> Delay39/1
  bank3/1 -> [ct_in_d1_g]
  bank5/1 -> bank3/1, bank7/1
  bank4/1 -> bank2/1, bank6/1
  bank2/1 -> [ct_in_d0_g]
  [sync256] -> [ct_in_sync_g]
  [dv256] -> [ct_in_dv_g]
  [d256] -> bank4/1, bank5/1
  make_interleaved_freqs/1(freq_id) -> we_delay33/1(d)
  we_delay33/1(q) -> freq_id/1
  Constant17/1 -> [obuf_trig_lower]
  Constant16/1 -> [obuf_trig_upper]
  [hmc_sync] -> [hmc_sync_g]
  bank1/1 -> Terminator1/1  "ZEN_wrdata"
  last_tag2/1 -> Logical12/2, we_delay15/1(d), [rd_addr_arm_raw]
  we_delay32/1(q) -> we_delay20/1(d)
  we_delay31/1(q) -> we_delay19/1(d)
  we_delay21/1(q) -> we_delay18/1(d)
  we_delay13/1(q) -> we_delay16/1(d)
  [dv256] -> Relational1/3
  Constant8/1 -> Concat2/1
  Constant6/1 -> Concat1/1
  Concat2/1 -> [wr_addr]
  hmc_addr_opt/1(" addr_opt") -> Concat2/2
  we_delay26/1(q) -> hmc_addr_opt/1(addr), [wr_addr_raw]
  in_sync/1 -> Delay36/1, tvg_data_gen_oneshot/1(sync), tvg_data_tone_gen/1(sync), tvg_data_gen/1(sync)  "sync128"
  in_dv/1 -> tvg_data_tone_gen/2(dv), tvg_data_gen/2(dv), Delay33/1, tvg_data_gen_oneshot/2(dv)  "dv128"
  prev_word/1 -> Concat3/1
  Mux3/1 -> Concat3/2, prev_word/1, [qt_d128_g]  "data128"
  Concat3/1 -> Delay14/1
  Logical2/1 -> Register/2
  Register/1 -> Logical3/1
  Logical3/1 -> Delay42/1, Logical9/1, Logical2/2
  [sync256] -> waddr/1
  [dv256] -> waddr/2
  waddr/1 -> [wr_addr_cnt], we_delay13/1(d)  "waddr_cnt"
  bank/1 -> Inverter3/1  "wrbank"
  spectrum_ctr/1 -> Terminator16/1  "wrspecctr"
  [wr_addr_cnt] -> spectrum_ctr1/1, bank/1, spectrum_ctr/1  "waddr"
  rd_addr_ctr/1 -> we_delay14/1(d)
  [rd_now] -> rd_addr_ctr/1
  Logical12/1 -> we_delay17/1(d), rd_addr_ctr/2
  Slice1/1 -> we_delay22/1(d)  "ZEN_tag_input"
  we_delay22/1(q) -> [rd_tag]  "zen_rdtag"
  [sync256] -> last_tag2/2
  [rd_now] -> last_tag2/1, last_tag2/3
  we_delay25/1(q) -> [rd_en]  "zen_rden"
  Constant/1 -> Relational1/1
  Relational1/1 -> edge_detect2/1(in)
  spectrum_ctr1/1 -> Relational1/2
  edge_detect2/1(out) -> [rd_now]  "rd_now"
  Inverter3/1 -> [rd_bank]  "rdbank"
  Delay1/1 -> Delay15/1
  [init_done] -> Logical9/2
  [postokay] -> Logical9/3
  Logical9/1 -> [dv256]  "dv_256"
  Delay14/1 -> [d256]  "d256"
  Delay15/1 -> [sync256]  "sync256"
  we_delay23/1(q) -> [rd_addr_raw]
  we_delay24/1(q) -> [rd_addr_arm]
  [dv256] -> Logical12/1
  Concat/1 -> we_delay23/1(d), Slice1/1, read_map_gen_interleave/1(addr)  "ZEN_addr_input"
  read_map_gen_interleave/1(" read_addr") -> hmc_addr_opt1/1(addr)
  Concat1/1 -> [rd_addr]
  we_delay16/1(q) -> we_delay26/1(d)  "ZEN_wrctr"
  [ct_tvg_en] -> Mux3/1
  in_d128/1 -> Delay34/1
  Delay35/1 -> Logical2/1, prev_word/2, Delay1/1, [qt_sync_g]
  Delay39/1 -> prev_word/3, Logical3/2, Register/3, Register/1, [qt_dv_g]
  we_delay17/1(q) -> we_delay25/1(d)  "ZEN_en_input"
  we_delay14/1(q) -> Concat/2  "ZEN_addr_ctr"
  we_delay15/1(q) -> we_delay24/1(d)  "ZEN_arm"
  [dv256] -> we_delay32/1(d)
  [d256] -> we_delay31/1(d)
  [sync256] -> we_delay21/1(d)
  we_delay18/1(q) -> we_delay27/1(d)
  we_delay19/1(q) -> bank1/1, we_delay28/1(d)
  we_delay20/1(q) -> we_delay29/1(d)  "ZEN_wr_dv"
  we_delay27/1(q) -> [wr_sync]
  we_delay28/1(q) -> [wr_d256]
  we_delay29/1(q) -> [wr_dv], [hmc_wr_dv_g]
  [ct_num_xeng] -> read_map_gen_interleave/2(num_x)
  [ct_num_xeng_recip] -> read_map_gen_interleave/3(one_over_num_x)
  [ct_chans_per_x] -> read_map_gen_interleave/4(chans_per_x_div8)
  hmc_addr_opt1/1(" addr_opt") -> Concat1/2
  [rd_bank] -> we_delay30/1(d)
  we_delay30/1(q) -> Concat/1  "ZEN_bank"
  Slice5/1 -> [hmc_d0_3]
  [p0f3] -> Slice5/1
  Slice4/1 -> [hmc_d0_2]
  [p0f2] -> Slice4/1
  Slice3/1 -> [hmc_d0_1]
  [p0f1] -> Slice3/1
  Slice2/1 -> [hmc_d0_0]
  [p0f0] -> Slice2/1, Slice6/1
  Slice/1 -> [hmc_out_p0f0_g]
  [p0f0] -> Slice/1
  [hmc_d256] -> bus_expand1/1(bus_in)
  bus_expand1/1(msb_out16) -> [p0f0]  "d256_f0"
  bus_expand1/2(out15) -> [p0f1]  "d256_f1"
  bus_expand1/3(out14) -> [p0f2]  "d256_f2"
  bus_expand1/4(out13) -> [p0f3]  "d256_f3"
  bus_expand1/5(out12) -> [p1f0]
  bus_expand1/6(out11) -> [p1f1]
  bus_expand1/7(out10) -> [p1f2]
  bus_expand1/8(out9) -> [p1f3]
  bus_expand1/9(out8) -> [p0f4]  "d256_f4"
  bus_expand1/10(out7) -> [p0f5]  "d256_f5"
  bus_expand1/11(out6) -> [p0f6]  "d256_f6"
  bus_expand1/12(out5) -> [p0f7]  "d256_f7"
  bus_expand1/13(out4) -> [p1f4]
  bus_expand1/14(out3) -> [p1f5]
  bus_expand1/15(out2) -> [p1f6]
  bus_expand1/16(lsb_out1) -> [p1f7]
  [p0f0] -> Concat4/1
  [p1f0] -> Concat4/2
  [p1f6] -> Concat12/2
  [p1f7] -> Concat10/2
  [p1f1] -> Concat5/2
  [p0f1] -> Concat5/1
  [p0f2] -> Concat6/1
  [p1f2] -> Concat6/2
  [p0f3] -> Concat7/1
  [p1f3] -> Concat7/2
  [p0f4] -> Concat8/1
  [p1f4] -> Concat8/2
  [p0f5] -> Concat9/1
  [p1f5] -> Concat9/2
  [p0f6] -> Concat12/1
  [p0f7] -> Concat10/1
  Concat4/1 -> [dbuf0]
  Concat5/1 -> [dbuf1]
  Concat6/1 -> [dbuf2]
  Concat7/1 -> [dbuf3]
  Concat8/1 -> [dbuf4]
  Concat9/1 -> [dbuf5]
  Concat12/1 -> [dbuf6]
  Concat10/1 -> [dbuf7]
  [dbuf1] -> Concat11/2
  [dbuf0] -> Concat11/1
  [dbuf2] -> Concat11/3
  [dbuf3] -> Concat11/4
  [dbuf4] -> Concat11/5
  [dbuf5] -> Concat11/6
  [dbuf6] -> Concat11/7
  [dbuf7] -> Concat11/8
  obuf/1(out_sync) -> we_delay12/1(d), make_interleaved_freqs/1(sync), [sync_ctrs_obuf_out]
  obuf/2(out_dv) -> we_delay10/1(d), make_interleaved_freqs/2(dv)
  obuf/3(out_d256) -> we_delay9/1(d)
  obuf/4(pkt_start) -> we_delay8/1(d)
  we_delay4/1(q) -> [sync_ctrs_obuf_in], [obuf_in_sync], obuf/1(in_sync)
  we_delay5/1(q) -> [obuf_in_dv], obuf/2(in_dv)
  we_delay6/1(q) -> [obuf_in_tag], obuf/3(in_tag)
  Concat11/1 -> [hmc_d256_reo]
  spectrum_ctr2/1 -> Concat13/1
  Mux/1 -> Concat13/2
  spectrum_ctr3/1 -> Concat13/3
  Concat13/1 -> we_delay7/1(d)
  we_delay7/1(q) -> obuf/4(in_d256)
  [hmc_tag] -> Mux/3
  spectrum_ctr4/1 -> Mux/2
  [hmc_d256_reo] -> spectrum_ctr4/1
  [ct_tag_insert_sel] -> Mux/1
  [hmc_d256_reo] -> we_delay11/1(d)
  [hmc_tag] -> we_delay1/1(d)
  [hmc_dv] -> we_delay2/1(d)
  [hmc_sync] -> we_delay3/1(d)
  we_delay11/1(q) -> spectrum_ctr3/1, spectrum_ctr2/1
  we_delay1/1(q) -> we_delay6/1(d)
  we_delay2/1(q) -> we_delay5/1(d)
  we_delay3/1(q) -> we_delay4/1(d)
  we_delay8/1(q) -> pkt_start/1
  we_delay9/1(q) -> out_d256/1
  we_delay10/1(q) -> out_dv/1
  we_delay12/1(q) -> out_sync/1
  hmc/2 -> convert_rd_en4/1
  hmc/1 -> Delay32/1  "hmc_d256"
  Delay32/1 -> [hmc_d256]
  Delay30/1 -> [hmc_dv]  "hmc_dv"
  Delay31/1 -> [hmc_tag]  "hmc_tag"
  convert_rd_en4/1 -> Delay30/1  "hmcout_dv"
  hmc/3 -> [hmc_wr_ready]
  hmc/4 -> [hmc_rd_ready]
  hmc/5 -> Delay31/1
  hmc/6 -> Terminator20/1
  hmc/7 -> Terminator21/1
  hmc/8 -> Terminator22/1
  hmc/9 -> Terminator23/1
  hmc/10 -> Terminator24/1
  hmc/11 -> [init_done]
  hmc/12 -> [postokay]
  Logical8/1 -> [ct_bank_error_g]  "same_bank"
  [rd_en_final_g] -> Logical10/2
  [wr_en_final_g] -> Logical10/1
  Logical10/1 -> Logical8/2
  Logical/1 -> Logical8/1
  Slice12/1 -> Logical/1  "final_wr_bank"
  Slice13/1 -> Logical/2  "final_rd_bank"
  [rd_addr_final_g] -> Slice13/1
  [wr_addr_final_g] -> Slice12/1
  [wr_d256] -> Delay18/1
  [wr_dv] -> Delay17/1
  [hmc_dv] -> [hmc_dv_g]
  [hmc_tag] -> [hmc_tag_g]
  [hmc_rd_ready] -> [hmc_rd_rdy_g]
  [hmc_wr_ready] -> [hmc_wr_rdy_g]
  Delay41/1 -> [hmc_postokay_g]
  Delay19/1 -> [hmc_init_done_g]
  [postokay] -> Delay41/1
  [init_done] -> Delay19/1
  Logical4/1 -> [hmc_err_rdrdy_g]
  [hmc_rd_ready] -> Inverter1/1
  [rd_en_final_g] -> Logical4/1
  Inverter1/1 -> Logical4/2
  [hmc_wr_ready] -> Inverter4/1
  Logical1/1 -> [hmc_err_wrrdy_g]  "err_wrrdy"
  Inverter4/1 -> Logical1/2
  [wr_en_final_g] -> Logical1/1
  Logical7/1 -> Logical5/1, Logical11/1
  [postokay] -> Logical7/2
  [init_done] -> Logical7/1
  Constant7/1 -> hmc/8
  Delay38/1 -> [rd_tag_final_g], hmc/6
  Delay37/1 -> [rd_addr_final_g], hmc/5
  Delay24/1 -> [wr_data_final_g], hmc/3
  Delay20/1 -> [wr_addr_final_g], hmc/2
  Constant5/1 -> hmc/10
  Constant2/1 -> hmc/11
  Delay9/1 -> Logical11/2  "RD_en"
  Logical11/1 -> [rd_en_final_g], hmc/4
  Delay13/1 -> Logical5/2  "WR_en"
  Logical5/1 -> [wr_en_final_g], hmc/1
  Delay18/1 -> Delay8/1
  Delay17/1 -> Delay13/1
  Constant4/1 -> hmc/12
  Constant3/1 -> hmc/9
  Constant1/1 -> hmc/7
  Delay11/1 -> Delay37/1  "RD_rdaddr"
  Delay8/1 -> Delay24/1
  Delay5/1 -> Delay20/1  "WR_addr"
  Delay12/1 -> Delay38/1  "RD_tag"
  [rd_en] -> Delay21/1
  [rd_addr] -> Delay22/1
  [rd_tag] -> Delay23/1
  [wr_en_final_g] -> Logical6/1
  [rd_en_final_g] -> Inverter/1
  Inverter/1 -> Logical6/2
  [wr_en_final_g] -> Inverter5/1
  [rd_en_final_g] -> Logical13/2
  Inverter5/1 -> Logical13/1
  Logical6/1 -> Logical14/1  "WR_SE_ERR"
  Logical14/1 -> [ct_en_sync_error_g], Inverter2/1
  Inverter2/1 -> Assertion/1  "SE_ERR"
  Logical13/1 -> Logical14/2  "RD_SE_ERR"
  [wr_addr_raw] -> Delay6/1
  Delay2/1 -> Delay3/1  "WR_raw_addr"
  Delay3/1 -> [wr_addr_raw_g]
  [wr_sync] -> Delay10/1
  Delay4/1 -> Delay40/1  "WR_sync"
  Delay6/1 -> Delay2/1
  [wr_addr] -> Delay7/1
  Delay7/1 -> Delay5/1
  Delay10/1 -> Delay4/1
  [rd_addr_raw] -> Delay25/1
  Delay16/1 -> Delay29/1  "RD_raw_addr"
  Delay21/1 -> Delay9/1
  Delay22/1 -> Delay11/1
  Delay23/1 -> Delay12/1
  Delay25/1 -> Delay16/1
  [rd_addr_arm] -> Delay26/1
  Delay26/1 -> Delay27/1
  Delay27/1 -> Delay28/1
  [rd_arm_final_g] -> Logical6/3
  Delay28/1 -> [rd_arm_final_g]
  Delay29/1 -> [rd_addr_raw_final_g]
  [tvgtone_p0] -> tvg_data_tone_gen/3(target0)
  [tvgtone_p1] -> tvg_data_tone_gen/4(target1)
  [tvgtone_levels] -> tvg_data_tone_gen/5(levels)
  Delay34/1 -> Mux3/2
  tvg_data_tone_gen/1(d128) -> Mux3/3
  Delay42/1 -> [hmc_dv]
